simulink model "sssc"  (Simulink 7.3)
settings: Solver=ode45  StartTime=0.0  StopTime=0.1  RelTol=1e-3
libraries: powerlib x14, powerlib_extras x1
settings Model: Creator=ayyapa  LastModifiedBy=Sree
settings OptimizationCC: InitFltsAndDblsToZero=on
settings DebuggingCC: SaveWithParameterizedLinksMsg=none  SignalResolutionControl=TryResolveAllWithWarning  MultiTaskDSMMsg=warning  MultiTaskCondExecSysMsg=none
settings RTWCC: IncludeERTFirstTime=on
settings GRTTargetCC: TargetFcnLib=ansi_tfl_tmw.mat

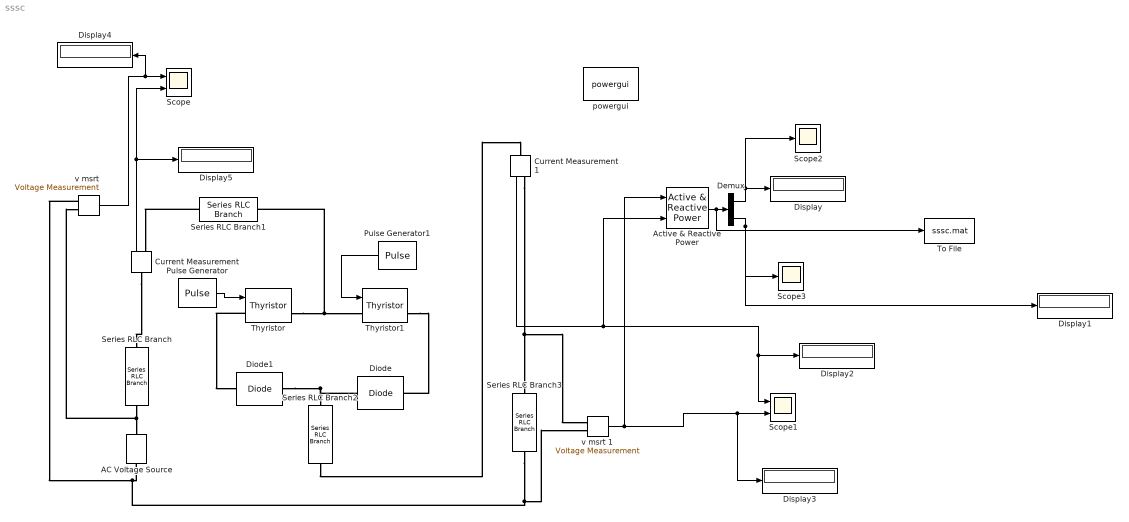
== system sssc ==
  AC Voltage Source : powerlib/Electrical Sources/AC Voltage Source  DialogController=POWERSYS.PowerSysDialog  SystemSampleTime=-1  Amplitude=11000  Phase=0  Frequency=50  SampleTime=0  Measurements=None
  Active & Reactive Power : powerlib_extras/Measurements/Active & Reactive Power  DialogController=POWERSYS.PowerSysDialog  SystemSampleTime=-1  f1=60
  Current Measurement : powerlib/Measurements/Current Measurement  DialogController=POWERSYS.PowerSysDialog  SystemSampleTime=-1  PhasorSimulation=off  OutputType=Complex  PSBequivalent=0
  Current Measurement1 : powerlib/Measurements/Current Measurement  DialogController=POWERSYS.PowerSysDialog  SystemSampleTime=-1  PhasorSimulation=off  OutputType=Complex  PSBequivalent=0
  Demux : Demux  Outputs=2
  Diode : powerlib/Power Electronics/Diode  DialogController=POWERSYS.PowerSysDialog  SystemSampleTime=-1  Ron=0.001  Lon=0  Vf=0.8  IC=0  UseSnubber=off  Rs=500  Cs=250e-9  Measurements=off
  Diode1 : powerlib/Power Electronics/Diode  DialogController=POWERSYS.PowerSysDialog  SystemSampleTime=-1  Ron=0.001  Lon=0  Vf=0.8  IC=0  UseSnubber=off  Rs=500  Cs=250e-9  Measurements=off
  Display{,1..5} (6 alike) : Display
  Pulse Generator : DiscretePulseGenerator  PulseType=Time based  Amplitude=1  Period=2  PulseWidth=50  PhaseDelay=0.012  SampleTime=1
  Pulse Generator1 : DiscretePulseGenerator  PulseType=Time based  Amplitude=1  Period=2  PulseWidth=50  PhaseDelay=0.022  SampleTime=1
  Scope : Scope  NumInputPorts=2
      settings: YMin=-5~-5  YMax=5~5
  Scope1 : Scope  NumInputPorts=2
      settings: YMin=-5~-5  YMax=5~5
  Scope2 : Scope
      settings: TimeRange=0.2  YMin=-4000  YMax=4000  SaveName=ScopeData2
  Scope3 : Scope
      settings: SaveName=ScopeData3
  Series RLC Branch : powerlib/Elements/Series RLC Branch  DialogController=POWERSYS.PowerSysDialog  PhysicalDomain=powersysdomain  SubClassName=unknown  LeftPortType=p1  RightPortType=p1  LConnTagsString=__new0  RConnTagsString=__new0  BranchType=RL  Resistance=0.1  Inductance=0.001  SetiL0=off  InitialCurrent=0  Capacitance=1e-6  Setx0=off  InitialVoltage=0  Measurements=None
  Series RLC Branch1 : powerlib/Elements/Series RLC Branch  DialogController=POWERSYS.PowerSysDialog  PhysicalDomain=powersysdomain  SubClassName=unknown  LeftPortType=p1  RightPortType=p1  LConnTagsString=__new0  RConnTagsString=__new0  BranchType=RL  Resistance=5  Inductance=0.023  SetiL0=off  InitialCurrent=0  Capacitance=1e-6  Setx0=off  InitialVoltage=0  Measurements=None
  Series RLC Branch2 : powerlib/Elements/Series RLC Branch  DialogController=POWERSYS.PowerSysDialog  PhysicalDomain=powersysdomain  SubClassName=unknown  LeftPortType=p1  RightPortType=p1  LConnTagsString=__new0  RConnTagsString=__new0  BranchType=C  Resistance=1  Inductance=1e-3  SetiL0=off  InitialCurrent=0  Capacitance=250e-6  Setx0=off  InitialVoltage=0  Measurements=None
  Series RLC Branch3 : powerlib/Elements/Series RLC Branch  DialogController=POWERSYS.PowerSysDialog  PhysicalDomain=powersysdomain  SubClassName=unknown  LeftPortType=p1  RightPortType=p1  LConnTagsString=__new0  RConnTagsString=__new0  BranchType=RL  Resistance=1  Inductance=0.02  SetiL0=off  InitialCurrent=0  Capacitance=1e-6  Setx0=off  InitialVoltage=0  Measurements=None
  Thyristor : powerlib/Power Electronics/Thyristor  DialogController=POWERSYS.PowerSysDialog  SystemSampleTime=-1  Ron=0.001  Lon=0  Vf=0.8  IC=0  Rs=500  Cs=250e-9  Measurements=on
  Thyristor1 : powerlib/Power Electronics/Thyristor  DialogController=POWERSYS.PowerSysDialog  SystemSampleTime=-1  Ron=0.001  Lon=0  Vf=0.8  IC=0  Rs=500  Cs=250e-9  Measurements=on
  To File : ToFile  Filename=sssc.mat
  powergui : powerlib/powergui  Priority=1  SystemSampleTime=-1  SimulationMode=Continuous  SampleTime=50e-6  frequency=60  SPID=off  DisableSnubberDevices=off  DisableRonSwitches=off  DisableVfSwitches=off  SwTol=0  Interpol=off  frequencyindice=50  echomessages=off  HookPort=off  DisplayEquations=off  FunctionMessages=off  EnableUseOfTLC=off  x0status=blocks  RestoreLinks=warning  Frange=[0:2:500]  Ylog=off  Xlog=on  ShowGrid=off  save=off  variable=ZData  ZoomFFT=off  StartTime=0.0  cycles=1  DisplayStyle=1  fundamental=60  FreqAxis=off  MaxFrequency=1000  frequencyindicesteady=1  RmsSteady=1  display=off  Ts=0  methode=off
  "v msrt " : powerlib/Measurements/Voltage Measurement  DialogController=POWERSYS.PowerSysDialog  SystemSampleTime=-1  PhasorSimulation=off  OutputType=Complex  PSBequivalent=0
  v msrt 1 : powerlib/Measurements/Voltage Measurement  DialogController=POWERSYS.PowerSysDialog  SystemSampleTime=-1  PhasorSimulation=off  OutputType=Complex  PSBequivalent=0
  wires:
  Current Measurement/1 -> Scope/2, Display5/1
  "v msrt "/1 -> Scope/1, Display4/1
  Pulse Generator1/1 -> Thyristor1/1
  Pulse Generator/1 -> Thyristor/1
  v msrt 1/1 -> Active & Reactive Power/1, Scope1/2, Display3/1
  Current Measurement1/1 -> Active & Reactive Power/2, Scope1/1, Display2/1
  Active & Reactive Power/1 -> Demux/1, To File/1
  Demux/1 -> Display/1, Scope2/1
  Demux/2 -> Display1/1, Scope3/1
  connections:
  Series RLC Branch/RConn1 -- AC Voltage Source/RConn1 -- "v msrt "/LConn2
  Series RLC Branch3/RConn1 -- "v msrt "/LConn1 -- AC Voltage Source/LConn1 -- v msrt 1/LConn2
  Current Measurement/LConn1 -- Series RLC Branch/LConn1
  Series RLC Branch1/RConn1 -- Current Measurement/RConn1
  Thyristor/RConn1 -- Thyristor1/LConn1 -- Series RLC Branch1/LConn1
  Thyristor/LConn1 -- Diode1/RConn1
  Thyristor1/RConn1 -- Diode/LConn1
  Diode1/LConn1 -- Series RLC Branch2/LConn1 -- Diode/RConn1
  Current Measurement1/RConn1 -- Series RLC Branch3/LConn1 -- v msrt 1/LConn1
  Series RLC Branch2/RConn1 -- Current Measurement1/LConn1
